simulink model "zynqRadioWLAN80211BeaconRxFPGAAD9361AD9364SL"  (R2016a)
settings: Solver=FixedStepDiscrete  SolverMode=SingleTasking  StartTime=0.0  StopTime=inf  RelTol=1e-3
PreLoadFcn:
  | load('commwlan80211BusTypes')
  | openMPDUGUI = true;
PostLoadFcn:
  | zynqRadioWLAN80211BeaconRxFPGAAD9361AD9364SL_params('init')
  | zynqRadioWLAN80211BeaconRxFPGAAD9361AD9364SL_params('scope')
InitFcn:
  | load('commwlan80211BusTypes')
  | openMPDUGUI = true;
  | mpduFigPos= [ 100 100 400 500];
model workspace: external: MAT-File (data not in the file)
undefined symbols (not defined in the file or in its folder): F, p80211, p80211hdl
libraries: simulink x11, hdlsllib x4, commutil2 x3, commwlan80211BeaconLib x2, commdigbbndpm3 x1, commsequence2 x1, commcrc2 x1, dspstat3 x1, dspmlti4 x1, dspsigops x1, dspmathops x1, sdrzblksprivate x1
(part 1 of 2)
CloseFcn:
  | clear BeaconFrameBodyType BeaconMPDUType CapabilityType FrameCtrlType InfoElementType MPDUHeaderType p80211 commwlan80211TxFilt rcvd openMPDUGUI mpduFigPos p80211hdl Hd
  | hFig = findall(0, 'Type', 'figure', 'Name', '802.11 Beacon Frame');
  | if ishghandle(hFig)
  | close(hFig);
  | end
  | clear hFig
  | if (exist('ans')==1) && (iscell(ans) && (numel(ans) == 0))
  | clear ans
  | end
Description:
  | IEEE 802.11 WLAN Beacon Frame Receiver for Captured Data
  | 
  | This example shows how to process a captured beacon frame and display the
  | frame information.
settings Model: ModifiedByFormat=The MathWorks Inc.  SimulationMode=accelerator  ExtModeTrigDuration=100  Creator=The MathWorks, Inc.  LastModifiedBy=The MathWorks Inc.
settings DataIOCC: LimitDataPoints=on  SaveFormat=Array  SaveOutput=off  SignalLogging=off  DSMLogging=off  StateSaveName=tmp_raccel_xout
settings OptimizationCC: BlockReduction=off  ConditionallyExecuteInputs=off  DefaultParameterBehavior=Inlined  InlineInvariantSignals=on  ExpressionDepthLimit=2147483647  EfficientMapNaN2IntZero=off
settings DebuggingCC: ReadBeforeWriteMsg=DisableAll  WriteAfterWriteMsg=DisableAll  WriteAfterReadMsg=DisableAll  AlgebraicLoopMsg=error  UnderspecifiedInitializationDetection=Classic  MergeDetectMultiDrivingBlocksExec=none  SolverPrmCheckMsg=warning  InheritedTsInSrcMsg=none  SingleTaskRateTransMsg=error  IntegerOverflowMsg=none  ParameterDowncastMsg=none  ParameterOverflowMsg=none  ParameterPrecisionLossMsg=none  ParameterTunabilityLossMsg=none  UniqueDataStoreMsg=error  AllowSymbolicDim=off  ModelReferenceDataLoggingMessage=none  StateNameClashWarn=warning  IntegerSaturationMsg=none
settings HardwareCC: ProdBitPerPointer=32  ProdLargestAtomicFloat=None  ProdIntDivRoundTo=Undefined  ProdEndianess=Unspecified  ProdWordSize=32  ProdHWDeviceType=ASIC/FPGA->ASIC/FPGA  TargetBitPerPointer=64  TargetLongLongMode=on  TargetIntDivRoundTo=Zero  TargetEndianess=LittleEndian  TargetWordSize=64  TargetHWDeviceType=MATLAB Host  ProdEqTarget=off
settings ModelReferenceCC: PropagateSignalLabelsOutOfModel=off
settings RTWCC: SystemTargetFile=raccel.tlc  TemplateMakefile=raccel_default_tmf  RTWVerbose=off  RTWUseSimCustomCode=on
settings CodeAppCC: GenerateComments=off  MaxIdLength=128  MangleLength=10  SimulinkBlockComments=off
settings RaccelTargetCC: ERTMultiwordTypeDef=System defined  ERTMultiwordLength=256  ParMdlRefBuildCompliant=off  GeneratePreprocessorConditionals=Disable all  ERTFirstTimeCompliant=off  MultiInstanceERTCode=off  ENABLE_SLEXEC_SSBRIDGE=0  RTWCAPISignals=off  RTWCAPIParams=off
settings ConfigComp: CovModelRefEnable=Off  CovSFcnEnable=off

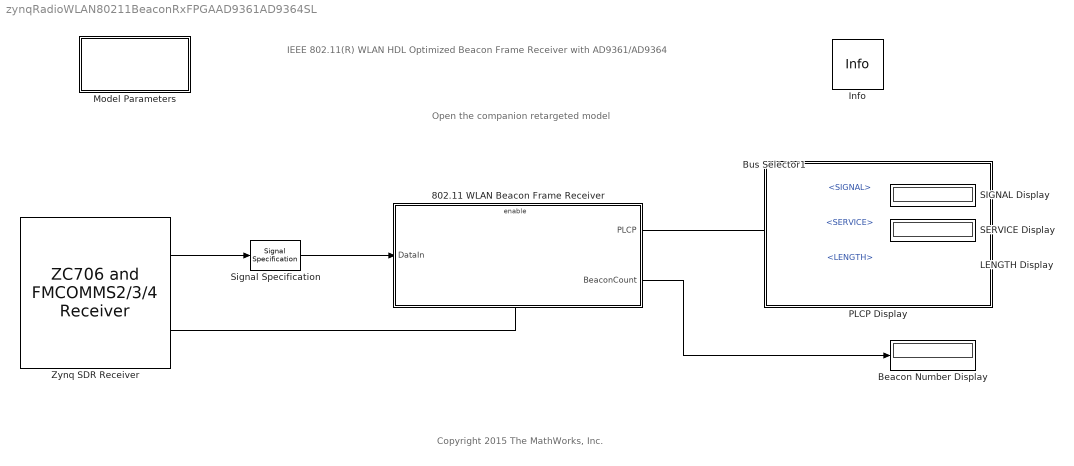
== system zynqRadioWLAN80211BeaconRxFPGAAD9361AD9364SL ==
  note: IEEE 802.11(R) WLAN
      | HDL Optimized Beacon Frame Receiver with AD9361/AD9364
  note: Copyright 2015 The MathWorks, Inc.
  note: Open the companion retargeted model
  802.11 WLAN Beacon Frame Receiver : Subsystem
  Beacon Number Display : Display
  Bus Selector1 : BusSelector  OutputSignals=SIGNAL,SERVICE,LENGTH
  Info : sdrzblksprivate/Info  SystemSampleTime=-1
  LENGTH Display : Display
  Model Parameters : Subsystem  mask(Model Parameters){chanNum=1, rfGain=30, rfFreqOffset=0, agcLoopGain=0.05, agcMaxGain=400, corrThreshold=1400}
      mask prompts: chanNum "Channel number"; rfGain "RF board gain:"; rfFreqOffset "RF center frequency offset:"; agcLoopGain "AGC loop gain:"; agcMaxGain "Maximum AGC gain:"; corrThreshold "Synchronization threshold:"
      mask help:
      | Choose 802.11 receiver parameters.
      |
      | You can select channel number for the 802.11 signals. You can set the AGC parameters and samples per chip used in the receiver. You can also set the synchronization threshold value to determine the correlation threshold used to declare the presence of an 802.11 packet.
      mask init:
      | zynqRadioWLAN80211BeaconRxFPGAAD9361AD9364SL_params('init', ...
      |     'ChannelNumber',   chanNum, ...
      |     'AGCLoopGain',     agcLoopGain, ...
      |     'AGCMaxGain',      agcMaxGain, ...
      |     'CorrThreshold',   corrThreshold, ...
      |     'RadioGain',       rfGain, ...
      |     'RadioFreqOffset', rfFreqOffset ...
      |     );
      mask TypeOptions chanNum: 1 | 2 | 3 | 4 | 5 | 6 | 7 | 8 | 9 | 10 | 11
      mask Display: disp('Model\nParameters')
  PLCP Display : Subsystem
      mask Display: disp('')
  SERVICE Display : Display
      settings: Format=hex (Stored Integer)
  SIGNAL Display : Display
      settings: Format=hex (Stored Integer)
  Signal Specification : SignalSpecification  SampleTime=p80211.RadioFrameLength/p80211.RadioBasebandRate
  Zynq SDR Receiver : zc706fmc234_lib/ZC706 and  FMCOMMS2//3//4  Receiver  IPAddress=192.168.3.2  CenterFrequencySource=Dialog  CenterFrequency=2.412e9+(p80211.ChannelNumber-1)*5e6+p80211.RadioFreqOffset  GainSource=Dialog  Gain=p80211.RadioGain  ChannelMapping=1  BasebandSampleRate=p80211.RadioBasebandRate  EnableBurstMode=on  NumFramesInBurst=p80211.RadioNumFramesInBurst  OutputDataType=int16  SamplesPerFrame=p80211.RadioFrameLength  LostSamplesOutputPort=off  RSSIOutputPort=off  DMATimeoutValue=1  blockMode=Normal  EnableQuadratureTracking=on  EnableRFDCTracking=on  EnableBasebandDCTracking=on  BypassUserLogic=on  ShowAdvancedProperties=on  ShowInternalProperties=off  subDeviceList=zynqReceiver  sdrExecutionMode=HW  dataUDPPort=-1  ctrlUDPPort=-1  SourceSelect=RF data  SourceConfiguration1=1023  FIRCoefficientSize=[ 128; 128 ]  FIRCoefficients=[ 111, -87, 147, -127, -18, -286, -312, -555, -601, -722, -642, -555, -303, -66, 221, 393, 488, 403, 219, -74, -343, -550, -582, -450, -146, 221, 569, 759, 735, 463, 20, -487, -885, -1048, -883, -418, 243, 897, 1340, 1394, 1002, 228, -715, -1549, -1980, -1819, -1028, 217, 1583, 2635, 2980, 2377, 853, -1275, -3435, -4926, -5080, -3454, 40, 5065, 10903, 16581, 21085, 23573, 23573, 21085, 16581, 10903, 5065, 40, -3454, -5080, -4926, -3435, -1275, 853, 2377, 2980, 2635, 1583, 217, -1028, -1819, -1980, -1549, -715, 228, 1002, 1394, 1340, 897, 243, -418, -883, -1048, -885, -487, 20, 463, 735, 759, 569, 221, -146, -450, -582, -550, -343, -74, 219, 403, 488, 393, 221, -66, -303, -555, -642, -722, -601, -555, -312, -286, -18, -127, 147, -87, 111; 382, -200, 711, -41, 645, 36, 346, -194, -119, -543, -472, -646, -404, -312, 45, 197, 413, 346, 241, -93, -373, -680, -755, -689, -356, 51, 515, 795, 870, 609, 136, -488, -1009, -1303, -1191, -712, 69, 885, 1516, 1692, 1336, 468, -662, -1740, -2378, -2329, -1494, -55, 1620, 2995, 3584, 3045, 1368, -1121, -3755, -5708, -6156, -4542, -710, 4969, 11669, 18243, 23486, 26391, 26391, 23486, 18243, 11669, 4969, -710, -4542, -6156, -5708, -3755, -1121, 1368, 3045, 3584, 2995, 1620, -55, -1494, -2329, -2378, -1740, -662, 468, 1336, 1692, 1516, 885, 69, -712, -1191, -1303, -1009, -488, 136, 609, 870, 795, 515, 51, -356, -689, -755, -680, -373, -93, 241, 346, 413, 197, 45, -312, -404, -646, -472, -543, -119, -194, 346, 36, 645, -41, 711, -200, 382 ]  FIRGain=[ 0; -12 ]  FIRDecimInterpFactor=[ 4; 4 ]  AnalogFilterCutoff=[ 2560000; 2560000 ]  FilterPathRates=[ 737280000, 184320000, 61440000, 30720000, 15360000, 3840000; 737280000, 184320000, 61440000, 30720000, 15360000, 3840000 ]  FilterDesignTypeForTx=DefaultFilterFromOther  FilterDesignTypeForRx=DefaultFilter  BISTLoopbackConfig=No Loopback  BISTPRBSMode=PRBS Disable  BISTToneMode=Tone Disable  BISTToneFrequency=F/32  BISTToneLevel=-6  BISTChannelMask=0  DataIsComplex=on  SimulateUsing=Code generation
  wires:
  802.11 WLAN Beacon Frame Receiver/1(PLCP) -> Bus Selector1/1
  Bus Selector1/3 -> LENGTH Display/1  "<LENGTH>"
  Bus Selector1/1 -> SIGNAL Display/1  "<SIGNAL>"
  Bus Selector1/2 -> SERVICE Display/1  "<SERVICE>"
  Zynq SDR Receiver/1 -> Signal Specification/1
  Zynq SDR Receiver/2 -> 802.11 WLAN Beacon Frame Receiver/Enable
  Signal Specification/1 -> 802.11 WLAN Beacon Frame Receiver/1(DataIn)
  802.11 WLAN Beacon Frame Receiver/2(BeaconCount) -> Beacon Number Display/1

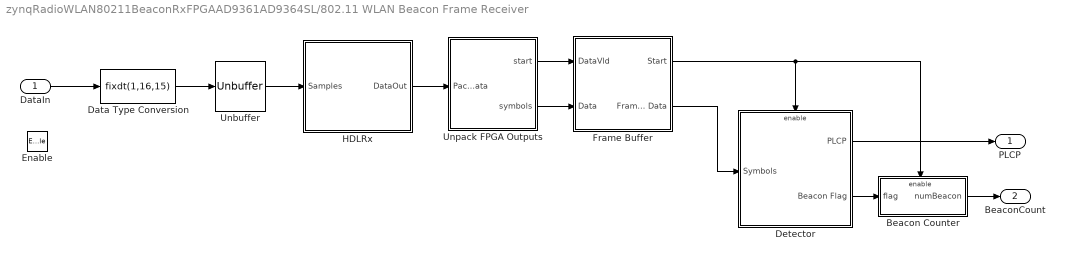
== system zynqRadioWLAN80211BeaconRxFPGAAD9361AD9364SL/802.11 WLAN Beacon Frame Receiver ==
  DataIn : Inport
  Enable : EnablePort
  Beacon Counter : Subsystem
  Data Type Conversion : DataTypeConversion  OutDataTypeStr=fixdt(1,16,15)  ConvertRealWorld=Stored Integer (SI)
  Detector : Subsystem
      settings: CloseFcn=clear BeaconFrameBodyType rcvd
  Frame Buffer : Subsystem
  HDLRx : Subsystem
  Unbuffer : Unbuffer  SampleBasedProcessing=Same as frame based
  Unpack FPGA Outputs : Subsystem
  PLCP : Outport
  BeaconCount : Outport  Port=2
  wires:
  Frame Buffer/1(Start) -> Detector/Enable, Beacon Counter/Enable
  Unbuffer/1 -> HDLRx/1(Samples)
  Frame Buffer/2(Framed Data) -> Detector/1(Symbols)
  Beacon Counter/1(numBeacon) -> BeaconCount/1
  Data Type Conversion/1 -> Unbuffer/1
  Detector/1(PLCP) -> PLCP/1
  DataIn/1 -> Data Type Conversion/1
  Detector/2(Beacon Flag) -> Beacon Counter/1(flag)
  HDLRx/1(DataOut) -> Unpack FPGA Outputs/1(PackedData)
  Unpack FPGA Outputs/1(start) -> Frame Buffer/1(DataVld)
  Unpack FPGA Outputs/2(symbols) -> Frame Buffer/2(Data)

== system zynqRadioWLAN80211BeaconRxFPGAAD9361AD9364SL/Model Parameters ==

== system zynqRadioWLAN80211BeaconRxFPGAAD9361AD9364SL/PLCP Display ==

== system zynqRadioWLAN80211BeaconRxFPGAAD9361AD9364SL/802.11 WLAN Beacon Frame Receiver/Beacon Counter ==
  flag : Inport
  Enable : EnablePort
  MATLAB Function : MATLAB Function  TreatAsAtomicUnit=on
  numBeacon : Outport
  wires:
  MATLAB Function/1(numBeacon) -> numBeacon/1
  flag/1 -> MATLAB Function/1(beaconflag)

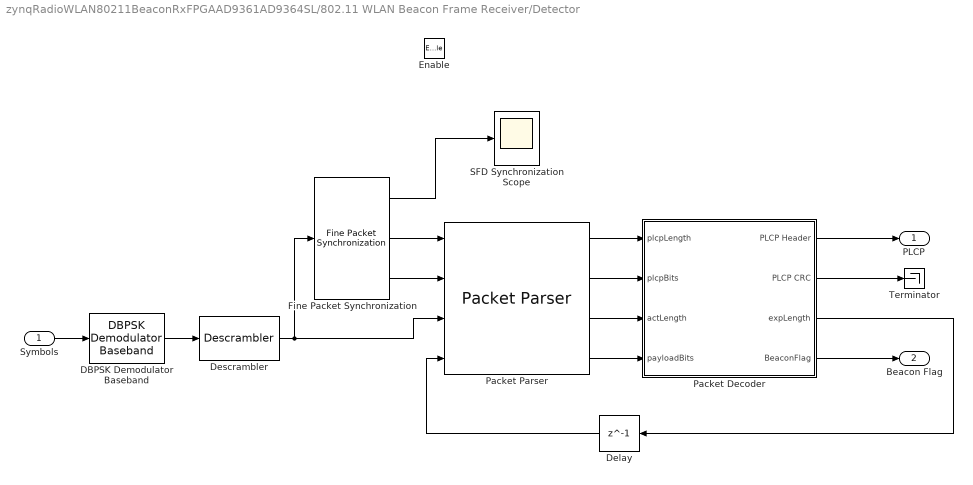
== system zynqRadioWLAN80211BeaconRxFPGAAD9361AD9364SL/802.11 WLAN Beacon Frame Receiver/Detector ==
  Symbols : Inport
  Enable : EnablePort  StatesWhenEnabling=reset  PropagateVarSize=During execution
  DBPSK Demodulator Baseband : commdigbbndpm3/DBPSK Demodulator Baseband  Ph=0  outDtype=uint32
  Delay : Delay  DelayLength=1  InitialCondition=0  InputProcessing=Columns as channels (frame based)
  Descrambler : commsequence2/Descrambler  M=2  poly=p80211.ScramblerPolynomial  iniStaSource=Dialog Parameter  ini_sta=[0 0 0 0 0 0 0]  resetViaPort=off
  Fine Packet Synchronization : commwlan80211BeaconLib/Fine Packet Synchronization
  Packet Decoder : Subsystem
  Packet Parser : commwlan80211BeaconLib/Packet Parser
  SFD Synchronization Scope : Scope
      settings: Priority=10
  Terminator : Terminator
  PLCP : Outport
  Beacon Flag : Outport  Port=2  InitialOutput=1
  wires:
  Fine Packet Synchronization/1 -> SFD Synchronization Scope/1
  DBPSK Demodulator Baseband/1 -> Descrambler/1
  Symbols/1 -> DBPSK Demodulator Baseband/1
  Descrambler/1 -> Fine Packet Synchronization/1, Packet Parser/3
  Fine Packet Synchronization/2 -> Packet Parser/1
  Fine Packet Synchronization/3 -> Packet Parser/2
  Delay/1 -> Packet Parser/4
  Packet Parser/2 -> Packet Decoder/2(plcpBits)
  Packet Parser/3 -> Packet Decoder/3(actLength)
  Packet Parser/4 -> Packet Decoder/4(payloadBits)
  Packet Decoder/1(PLCP Header) -> PLCP/1
  Packet Parser/1 -> Packet Decoder/1(plcpLength)
  Packet Decoder/2(PLCP CRC) -> Terminator/1
  Packet Decoder/3(expLength) -> Delay/1
  Packet Decoder/4(BeaconFlag) -> Beacon Flag/1

== system zynqRadioWLAN80211BeaconRxFPGAAD9361AD9364SL/802.11 WLAN Beacon Frame Receiver/Frame Buffer ==
  DataVld : Inport
  Data : Inport  Port=2
  Buffer1 : Buffer  N=128  TreatMby1Signals=One channel  OutputFrames=off
  Buffer2 : Buffer  N=128  TreatMby1Signals=One channel  OutputFrames=off
  Data Type Conversion : DataTypeConversion
  Received Symbols : ConstellationDiagram  Tag=ScatterPlot  Priority=2
  data_framer : MATLAB Function  TreatAsAtomicUnit=on
  Start : Outport
  Framed Data : Outport  Port=2
  wires:
  Data Type Conversion/1 -> Framed Data/1
  data_framer/2(framed_data) -> Data Type Conversion/1
  data_framer/1(RxGo) -> Start/1
  Buffer1/1 -> data_framer/2(data), Received Symbols/1
  DataVld/1 -> Buffer2/1
  Data/1 -> Buffer1/1
  Buffer2/1 -> data_framer/1(datavld)

== system zynqRadioWLAN80211BeaconRxFPGAAD9361AD9364SL/802.11 WLAN Beacon Frame Receiver/HDLRx ==
  Samples : Inport
  FPGA to Host : Subsystem
  HDLRx Controller : Subsystem
  HDLRx Front End : Subsystem
  DataOut : Outport
  wires:
  Samples/1 -> HDLRx Front End/1(Samples)
  HDLRx Controller/1(Start) -> FPGA to Host/1(start)
  HDLRx Front End/1(rcvd) -> HDLRx Controller/1(Rx Signal)
  HDLRx Controller/2(Symbols) -> FPGA to Host/2(symbol)
  FPGA to Host/1(Out) -> DataOut/1

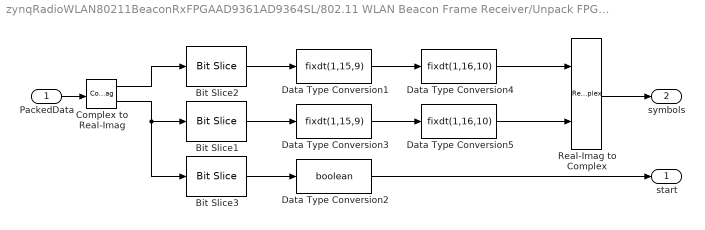
== system zynqRadioWLAN80211BeaconRxFPGAAD9361AD9364SL/802.11 WLAN Beacon Frame Receiver/Unpack FPGA Outputs ==
  PackedData : Inport
  Bit Slice1 : hdlsllib/HDL Operations/Bit Slice  lidx=15  ridx=1
  Bit Slice2 : hdlsllib/HDL Operations/Bit Slice  lidx=15  ridx=1
  Bit Slice3 : hdlsllib/HDL Operations/Bit Slice  lidx=0  ridx=0
  Complex to Real-Imag : ComplexToRealImag
  Data Type Conversion1 : DataTypeConversion  OutDataTypeStr=fixdt(1,15,9)  ConvertRealWorld=Stored Integer (SI)
  Data Type Conversion2 : DataTypeConversion  OutDataTypeStr=boolean
  Data Type Conversion3 : DataTypeConversion  OutDataTypeStr=fixdt(1,15,9)  ConvertRealWorld=Stored Integer (SI)
  Data Type Conversion4 : DataTypeConversion  OutDataTypeStr=fixdt(1,16,10)
  Data Type Conversion5 : DataTypeConversion  OutDataTypeStr=fixdt(1,16,10)
  Real-Imag to Complex : RealImagToComplex
  start : Outport
  symbols : Outport  Port=2
  wires:
  PackedData/1 -> Complex to Real-Imag/1
  Real-Imag to Complex/1 -> symbols/1
  Complex to Real-Imag/1 -> Bit Slice2/1
  Complex to Real-Imag/2 -> Bit Slice3/1, Bit Slice1/1
  Bit Slice3/1 -> Data Type Conversion2/1
  Data Type Conversion2/1 -> start/1
  Bit Slice2/1 -> Data Type Conversion1/1
  Bit Slice1/1 -> Data Type Conversion3/1
  Data Type Conversion1/1 -> Data Type Conversion4/1
  Data Type Conversion4/1 -> Real-Imag to Complex/1
  Data Type Conversion3/1 -> Data Type Conversion5/1
  Data Type Conversion5/1 -> Real-Imag to Complex/2

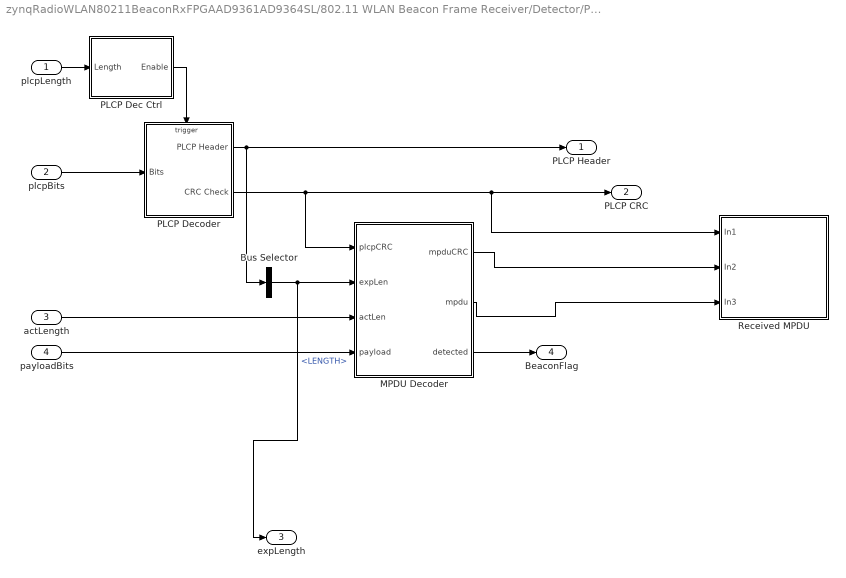
== system zynqRadioWLAN80211BeaconRxFPGAAD9361AD9364SL/802.11 WLAN Beacon Frame Receiver/Detector/Packet Decoder ==
  plcpLength : Inport
  plcpBits : Inport  Port=2
  actLength : Inport  Port=3
  payloadBits : Inport  Port=4
  Bus Selector : BusSelector  OutputSignals=LENGTH
  MPDU Decoder : MATLAB Function  TreatAsAtomicUnit=on
  PLCP Dec Ctrl : Subsystem
  PLCP Decoder : Subsystem
  Received MPDU : Subsystem  mask(MPDU GUI){OpenScopeAtSimStart=openMPDUGUI, figPosition=mpduFigPos}
      mask prompts: OpenScopeAtSimStart "Open GUI at start of simulation"; figPosition "Position"
      mask help: Display contents of the MPDU.
      mask Display: disp('MPDU GUI')
  PLCP Header : Outport
  PLCP CRC : Outport  Port=2
  expLength : Outport  Port=3
  BeaconFlag : Outport  Port=4
  wires:
  PLCP Dec Ctrl/1(Enable) -> PLCP Decoder/Trigger
  Bus Selector/1 -> MPDU Decoder/2(expLen), expLength/1  "<LENGTH>"
  PLCP Decoder/1(PLCP Header) -> Bus Selector/1, PLCP Header/1
  plcpLength/1 -> PLCP Dec Ctrl/1(Length)
  plcpBits/1 -> PLCP Decoder/1(Bits)
  actLength/1 -> MPDU Decoder/3(actLen)
  payloadBits/1 -> MPDU Decoder/4(payload)
  MPDU Decoder/1(mpduCRC) -> Received MPDU/2(In2)
  MPDU Decoder/2(mpdu) -> Received MPDU/3(In3)
  PLCP Decoder/2(CRC Check) -> MPDU Decoder/1(plcpCRC), Received MPDU/1(In1), PLCP CRC/1
  MPDU Decoder/3(detected) -> BeaconFlag/1

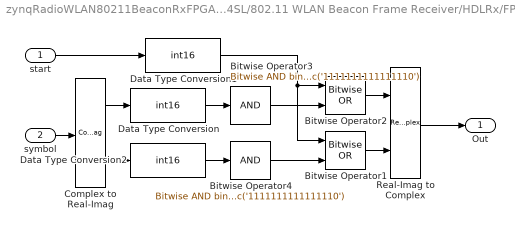
== system zynqRadioWLAN80211BeaconRxFPGAAD9361AD9364SL/802.11 WLAN Beacon Frame Receiver/HDLRx/FPGA to Host ==
  start : Inport
  symbol : Inport  Port=2
  Bitwise Operator1 : simulink/Logic and Bit Operations/Bitwise Operator  logicop=OR  UseBitMask=off  NumInputPorts=2  BitMask=bin2dec('11011001')  BitMaskRealWorld=Stored Integer
  Bitwise Operator2 : simulink/Logic and Bit Operations/Bitwise Operator  logicop=OR  UseBitMask=off  NumInputPorts=2  BitMask=bin2dec('11011001')  BitMaskRealWorld=Stored Integer
  Bitwise Operator3 : simulink/Logic and Bit Operations/Bitwise Operator  logicop=AND  UseBitMask=on  BitMask=bin2dec('1111111111111110')  BitMaskRealWorld=Stored Integer
  Bitwise Operator4 : simulink/Logic and Bit Operations/Bitwise Operator  logicop=AND  UseBitMask=on  BitMask=bin2dec('1111111111111110')  BitMaskRealWorld=Stored Integer
  Complex to Real-Imag : ComplexToRealImag
  Data Type Conversion : DataTypeConversion  OutDataTypeStr=int16  ConvertRealWorld=Stored Integer (SI)
  Data Type Conversion1 : DataTypeConversion  OutDataTypeStr=int16
  Data Type Conversion2 : DataTypeConversion  OutDataTypeStr=int16  ConvertRealWorld=Stored Integer (SI)
  Real-Imag to Complex : RealImagToComplex
  Out : Outport
  wires:
  symbol/1 -> Complex to Real-Imag/1
  start/1 -> Data Type Conversion1/1
  Bitwise Operator2/1 -> Real-Imag to Complex/1
  Bitwise Operator1/1 -> Real-Imag to Complex/2
  Real-Imag to Complex/1 -> Out/1
  Complex to Real-Imag/1 -> Data Type Conversion/1
  Complex to Real-Imag/2 -> Data Type Conversion2/1
  Data Type Conversion/1 -> Bitwise Operator3/1
  Data Type Conversion2/1 -> Bitwise Operator4/1
  Bitwise Operator4/1 -> Bitwise Operator1/2
  Bitwise Operator3/1 -> Bitwise Operator2/2
  Data Type Conversion1/1 -> Bitwise Operator1/1, Bitwise Operator2/1

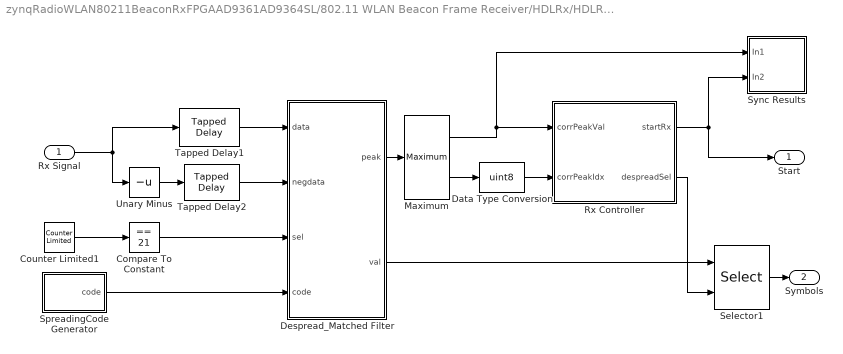
== system zynqRadioWLAN80211BeaconRxFPGAAD9361AD9364SL/802.11 WLAN Beacon Frame Receiver/HDLRx/HDLRx Controller ==
  Rx Signal : Inport
  Compare To Constant : simulink/Logic and Bit Operations/Compare To Constant  relop===  const=21  OutDataTypeStr=boolean
  Counter Limited1 : simulink/Sources/Counter Limited  uplimit=21  tsamp=-1
  Data Type Conversion : DataTypeConversion  OutDataTypeStr=uint8
  Despread_Matched Filter : Subsystem
  Maximum : dspstat3/Maximum  fcn=Value and Index  reset=None  InputProcessing=Columns as channels (frame based)  indexBase=One  operateOver=Each column  Dimension=1  operation=maximum  roiEnable=off  roiType=Rectangles  roiPortion=Entire ROI  roiOutput=Individual statistics for each ROI  roiFlag=off  accumDataTypeStr=Inherit: Same as product output  accumLastDataTypeStr=Inherit: Same as product output  roundingMode=Floor  overflowMode=off
  Rx Controller : MATLAB Function  TreatAsAtomicUnit=on
  Selector1 : Selector  InputPortWidth=22  IndexOptions=Index vector (port)  Indices=[1 3]  OutputSizes=1
  "SpreadingCode Generator " : Subsystem
  Sync Results : Subsystem
  Tapped Delay1 : simulink/Discrete/Tapped Delay  vinit=0  samptime=-1  NumDelays=21  DelayOrder=Newest  includeCurrent=on
  Tapped Delay2 : simulink/Discrete/Tapped Delay  vinit=0  samptime=-1  NumDelays=21  DelayOrder=Newest  includeCurrent=on
  Unary Minus : UnaryMinus
  Start : Outport
  Symbols : Outport  Port=2
  wires:
  Compare To Constant/1 -> Despread_Matched Filter/3(sel)
  Despread_Matched Filter/2(val) -> Selector1/1
  Despread_Matched Filter/1(peak) -> Maximum/1
  Rx Signal/1 -> Tapped Delay1/1, Unary Minus/1
  Tapped Delay1/1 -> Despread_Matched Filter/1(data)
  Selector1/1 -> Symbols/1
  Rx Controller/2(despreadSel) -> Selector1/2
  Maximum/1 -> Sync Results/1(In1), Rx Controller/1(corrPeakVal)
  Counter Limited1/1 -> Compare To Constant/1
  Unary Minus/1 -> Tapped Delay2/1
  Tapped Delay2/1 -> Despread_Matched Filter/2(negdata)
  Maximum/2 -> Data Type Conversion/1
  Data Type Conversion/1 -> Rx Controller/2(corrPeakIdx)
  Rx Controller/1(startRx) -> Start/1, Sync Results/2(In2)
  "SpreadingCode Generator "/1(code) -> Despread_Matched Filter/4(code)

== system zynqRadioWLAN80211BeaconRxFPGAAD9361AD9364SL/802.11 WLAN Beacon Frame Receiver/HDLRx/HDLRx Front End ==
  note: AGC implements the square law method:
      | e(n) = R - abs(x(n))^2;  % R = 1;
      | g(n) = g(n-1) + K*e(n);
  note: |U|^2 = re(u)^2+im(u)^2
  Samples : Inport
  AGC : Subsystem
  AGC Results : Subsystem
  Coarse Frequency Compensation : Subsystem
  Delay3 : Delay  DelayLength=1  InitialCondition=0
  Frequency Offset : Scope
  Inputreg : Delay  DelayLength=1  InitialCondition=0
  RCFilter : Subsystem
  rcvd : Outport
  wires:
  AGC/2(gain) -> AGC Results/2(In2)
  RCFilter/1(Out1) -> Delay3/1
  Samples/1 -> Inputreg/1
  Inputreg/1 -> RCFilter/1(In1)
  Delay3/1 -> AGC/1(x), AGC Results/3(In3)
  AGC/1(y) -> Coarse Frequency Compensation/1(x), AGC Results/1(In1)
  Coarse Frequency Compensation/1(y) -> rcvd/1
  Coarse Frequency Compensation/2(offset) -> Frequency Offset/1

== system zynqRadioWLAN80211BeaconRxFPGAAD9361AD9364SL/802.11 WLAN Beacon Frame Receiver/Detector/Packet Decoder/PLCP Dec Ctrl ==
  Length : Inport
  Compare To Constant : simulink/Logic and Bit Operations/Compare To Constant  relop=>=  const=p80211.PLCPHeaderLength  OutDataTypeStr=uint8
  Enable : Outport
  wires:
  Length/1 -> Compare To Constant/1
  Compare To Constant/1 -> Enable/1

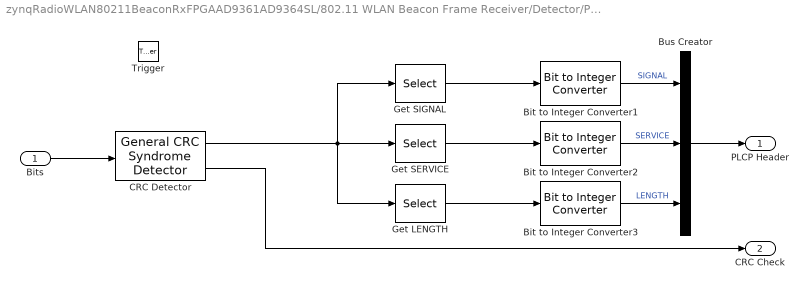
== system zynqRadioWLAN80211BeaconRxFPGAAD9361AD9364SL/802.11 WLAN Beacon Frame Receiver/Detector/Packet Decoder/PLCP Decoder ==
  Bits : Inport
  Trigger : TriggerPort  VariantControl=Variant  PortDimensions=1
  Bit to Integer Converter1 : commutil2/Bit to Integer Converter  nbits=8  bitOrder=LSB first  signedOutputValues=Unsigned  outDtype=Inherit via internal rule  outDtypeSigned=Inherit via internal rule
  Bit to Integer Converter2 : commutil2/Bit to Integer Converter  nbits=8  bitOrder=LSB first  signedOutputValues=Unsigned  outDtype=Inherit via internal rule  outDtypeSigned=Inherit via internal rule
  Bit to Integer Converter3 : commutil2/Bit to Integer Converter  nbits=16  bitOrder=LSB first  signedOutputValues=Unsigned  outDtype=uint16  outDtypeSigned=Inherit via internal rule
  Bus Creator : BusCreator  Inputs=3
  CRC Detector : commcrc2/General CRC Syndrome Detector  genPoly=[1 0 0 0 1 0 0 0 0 0 0 1 0 0 0 0 1]  iniStates=1  directMethod=on  reflectInputBytes=off  reflectChecksums=off  finalXOR=1  numChecksums=1
  Get LENGTH : Selector  InputPortWidth=32  IndexOptions=Index vector (dialog)  Indices=17:32  OutputSizes=1
  Get SERVICE : Selector  InputPortWidth=32  IndexOptions=Index vector (dialog)  Indices=9:16  OutputSizes=1
  Get SIGNAL : Selector  InputPortWidth=32  IndexOptions=Index vector (dialog)  Indices=1:8  OutputSizes=1
  PLCP Header : Outport
  CRC Check : Outport  Port=2
  wires:
  Bus Creator/1 -> PLCP Header/1
  Bit to Integer Converter3/1 -> Bus Creator/3  "LENGTH"
  Bits/1 -> CRC Detector/1
  Bit to Integer Converter2/1 -> Bus Creator/2  "SERVICE"
  Bit to Integer Converter1/1 -> Bus Creator/1  "SIGNAL"
  Get LENGTH/1 -> Bit to Integer Converter3/1
  Get SERVICE/1 -> Bit to Integer Converter2/1
  Get SIGNAL/1 -> Bit to Integer Converter1/1
  CRC Detector/1 -> Get SIGNAL/1, Get SERVICE/1, Get LENGTH/1
  CRC Detector/2 -> CRC Check/1

== system zynqRadioWLAN80211BeaconRxFPGAAD9361AD9364SL/802.11 WLAN Beacon Frame Receiver/Detector/Packet Decoder/Received MPDU ==
  In1 : Inport
  In2 : Inport  Port=2
  In3 : Inport  Port=3
  Received MPDU GUI : MATLAB Function  TreatAsAtomicUnit=on
  wires:
  In3/1 -> Received MPDU GUI/3(mpdu)
  In2/1 -> Received MPDU GUI/2(mpduCRC)
  In1/1 -> Received MPDU GUI/1(plcpCRC)

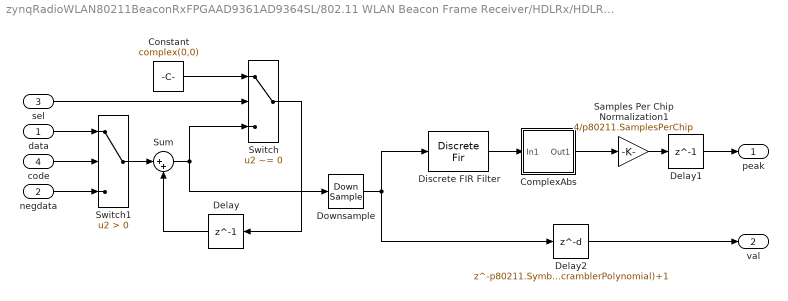
== system zynqRadioWLAN80211BeaconRxFPGAAD9361AD9364SL/802.11 WLAN Beacon Frame Receiver/HDLRx/HDLRx Controller/Despread_Matched Filter ==
  data : Inport
  negdata : Inport  Port=2
  sel : Inport  Port=3
  code : Inport  Port=4
  ComplexAbs : Subsystem
  Constant : Constant  Value=complex(0,0)  OutDataTypeStr=fixdt(1,16,7)  SampleTime=-1
  Delay : Delay  DelayLength=1  InitialCondition=0
  Delay1 : Delay  DelayLength=1  InitialCondition=0
  Delay2 : Delay  DelayLength=p80211.SymbolsPerChannelFrame-2+length(p80211.ScramblerPolynomial)+1  InitialCondition=0
  Discrete FIR Filter : DiscreteFir  Coefficients=fliplr(reshape(p80211hdl.syncsig128,1,128))  CoefDataTypeStr=fixdt(1,4,0)  ProductDataTypeStr=fixdt(1,16,3)  AccumDataTypeStr=fixdt(1,16,2)
  Downsample : DownSample  N=22  phase=21  RateOptions=Allow multirate processing
  Samples Per Chip Normalization1 : Gain  Gain=4/p80211.SamplesPerChip  OutDataTypeStr=Inherit: Same as input
  Sum : Sum  Inputs=|++  OutDataTypeStr=fixdt(1,16,8)  RndMeth=Round  SaturateOnIntegerOverflow=on
  Switch : Switch  Criteria=u2 ~= 0
  Switch1 : Switch  Criteria=u2 > Threshold
  peak : Outport
  val : Outport  Port=2
  wires:
  sel/1 -> Switch/2
  Switch1/1 -> Sum/1
  Samples Per Chip Normalization1/1 -> Delay1/1
  Discrete FIR Filter/1 -> ComplexAbs/1(In1)
  ComplexAbs/1(Out1) -> Samples Per Chip Normalization1/1
  Downsample/1 -> Delay2/1, Discrete FIR Filter/1
  Delay2/1 -> val/1
  Switch/1 -> Delay/1
  Constant/1 -> Switch/1
  code/1 -> Switch1/2
  Delay/1 -> Sum/2
  data/1 -> Switch1/1
  Sum/1 -> Switch/3, Downsample/1
  negdata/1 -> Switch1/3
  Delay1/1 -> peak/1

== system zynqRadioWLAN80211BeaconRxFPGAAD9361AD9364SL/802.11 WLAN Beacon Frame Receiver/HDLRx/HDLRx Controller/SpreadingCode Generator  ==
  Selector : Selector  InputPortWidth=22  IndexOptions=Index vector (dialog)  Indices=1  OutputSizes=1
  Signal Specification1 : SignalSpecification  OutDataTypeStr=fixdt(1,2,0)
  Tapped Delay : simulink/Discrete/Tapped Delay  vinit=p80211hdl.spreadingcode  samptime=-1  NumDelays=22  DelayOrder=Oldest  includeCurrent=off
  code : Outport
  wires:
  Selector/1 -> code/1, Signal Specification1/1
  Signal Specification1/1 -> Tapped Delay/1
  Tapped Delay/1 -> Selector/1

== system zynqRadioWLAN80211BeaconRxFPGAAD9361AD9364SL/802.11 WLAN Beacon Frame Receiver/HDLRx/HDLRx Controller/Sync Results ==
  In1 : Inport
  In2 : Inport  Port=2
  Buffer : Buffer  N=p80211.SamplesPerChannelFrame  TreatMby1Signals=One channel  OutputFrames=off
  Buffer1 : Buffer  N=128  TreatMby1Signals=One channel  OutputFrames=off
  Synchronization Scope : Scope  NumInputPorts=2
      settings: Priority=1
  wires:
  In1/1 -> Buffer/1
  In2/1 -> Buffer1/1
  Buffer/1 -> Synchronization Scope/1
  Buffer1/1 -> Synchronization Scope/2

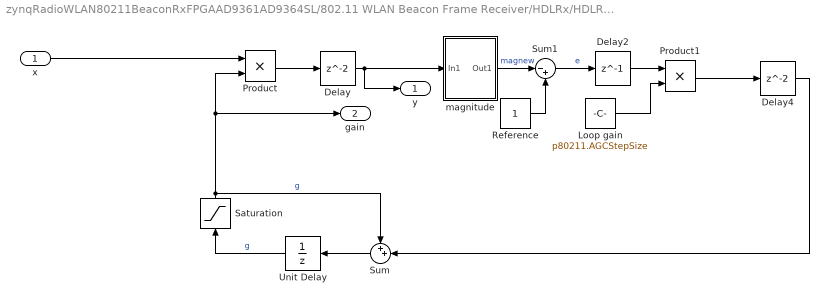
== system zynqRadioWLAN80211BeaconRxFPGAAD9361AD9364SL/802.11 WLAN Beacon Frame Receiver/HDLRx/HDLRx Front End/AGC ==
  x : Inport
  Delay : Delay  InitialCondition=0
  Delay2 : Delay  DelayLength=1  InitialCondition=0
  Delay4 : Delay  InitialCondition=0
  Loop gain : Constant  Value=p80211.AGCStepSize  OutDataTypeStr=fixdt(1,16,12)  SampleTime=-1
  Product : Product  OutDataTypeStr=fixdt(1,16,10)  SaturateOnIntegerOverflow=on
  Product1 : Product  OutDataTypeStr=fixdt(1,16,10)  SaturateOnIntegerOverflow=on
  Reference : Constant  OutDataTypeStr=fixdt(1,16,7)  SampleTime=-1
  Saturation : Saturate  UpperLimit=p80211.AGCUpperLimit  LowerLimit=1e-5  OutDataTypeStr=fixdt(1,16,6)
  Sum : Sum  Inputs=++|  OutDataTypeStr=fixdt(1,16,6)  SaturateOnIntegerOverflow=on
  Sum1 : Sum  Inputs=|-+  OutDataTypeStr=Inherit: Same as first input
  Unit Delay : UnitDelay  InitialCondition=1  SampleTime=-1
  magnitude : Subsystem
  y : Outport  PortDimensions=1
  gain : Outport  Port=2
  wires:
  x/1 -> Product/1
  Delay/1 -> y/1, magnitude/1(In1)
  Saturation/1 -> gain/1, Product/2, Sum/1  "g"
  Delay2/1 -> Product1/1
  Unit Delay/1 -> Saturation/1  "g"
  Loop gain/1 -> Product1/2
  Sum/1 -> Unit Delay/1
  Reference/1 -> Sum1/2
  Delay4/1 -> Sum/2
  magnitude/1(Out1) -> Sum1/1  "magnew"
  Product/1 -> Delay/1
  Product1/1 -> Delay4/1
  Sum1/1 -> Delay2/1  "e"

== system zynqRadioWLAN80211BeaconRxFPGAAD9361AD9364SL/802.11 WLAN Beacon Frame Receiver/HDLRx/HDLRx Front End/AGC Results ==
  In1 : Inport
  In2 : Inport  Port=2
  In3 : Inport  Port=3
  AGC Scope : Scope  NumInputPorts=3
  Buffer1 : Buffer  N=p80211.SamplesPerChannelFrame  TreatMby1Signals=One channel  OutputFrames=off
  Buffer2 : Buffer  N=p80211.SamplesPerChannelFrame  TreatMby1Signals=One channel  OutputFrames=off
  Buffer3 : Buffer  N=p80211.SamplesPerChannelFrame  TreatMby1Signals=One channel  OutputFrames=off
  ToFixPt1 : DataTypeConversion  OutDataTypeStr=double
  ToFixPt2 : DataTypeConversion  OutDataTypeStr=double
  wires:
  In3/1 -> Buffer1/1
  In2/1 -> Buffer2/1
  In1/1 -> Buffer3/1
  Buffer1/1 -> AGC Scope/1
  Buffer2/1 -> ToFixPt1/1
  Buffer3/1 -> ToFixPt2/1
  ToFixPt2/1 -> AGC Scope/3
  ToFixPt1/1 -> AGC Scope/2

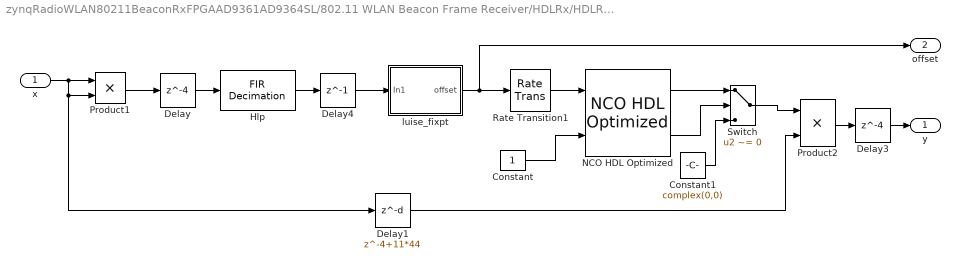
== system zynqRadioWLAN80211BeaconRxFPGAAD9361AD9364SL/802.11 WLAN Beacon Frame Receiver/HDLRx/HDLRx Front End/Coarse Frequency Compensation ==
  x : Inport  PortDimensions=1
  Constant : Constant  OutDataTypeStr=boolean  SampleTime=-1
  Constant1 : Constant  Value=complex(0,0)  OutDataTypeStr=fixdt(1,16,14)  SampleTime=-1
  Delay : Delay  DelayLength=4  InitialCondition=0
  Delay1 : Delay  DelayLength=4+11*44  InitialCondition=0
  Delay3 : Delay  DelayLength=4  InitialCondition=0
  Delay4 : Delay  DelayLength=1  InitialCondition=0
  Hlp : dspmlti4/FIR Decimation  Tag=BlockMethodSubSystem  FilterSource=Dialog parameters  h=Hd.Numerator  D=44  filtStruct=Direct form  FilterObject=Hd  framing=Allow multirate processing  inputOffset=0  outputBufInitCond=0  roundingMode=Floor  overflowMode=off  firstCoeffMode=Binary point scaling  firstCoeffWordLength=16  firstCoeffFracLength=15  firstCoeffDataTypeStr=fixdt(1,16,15)  firstCoeffMin=[]  firstCoeffMax=[]  firstCoeffLastDataTypeStr=fixdt(1,16,15)  prodOutputMode=Binary point scaling  prodOutputWordLength=32  prodOutputFracLength=20  prodOutputDataTypeStr=fixdt(1,32,20)  prodOutputLastDataTypeStr=fixdt(1,32,20)  accumDataTypeStr=Inherit: Same as product output  accumLastDataTypeStr=Inherit: Same as product output  outputMin=[]  outputMax=[]
  NCO HDL Optimized : dspsigops/NCO HDL Optimized  PhaseIncrementSource=Input port  PhaseIncrement=100  PhaseOffsetSource=Property  PhaseOffset=0  DitherSource=Property  NumDitherBits=4  PhaseQuantization=on  NumQuantizerAccumulatorBits=14  LUTCompress=on  ResetAction=off  ValidInputPort=on  Waveform=Complex exponential  PhasePort=off  AccumulatorWL=24  OutputDataType=Binary point scaling  OutputWL=16  OutputFL=14  SimulateUsing=Code generation
  Product1 : Product  OutDataTypeStr=fixdt(1,16,6)  RndMeth=Zero
  Product2 : Product  OutDataTypeStr=fixdt(1,16,10)  SaturateOnIntegerOverflow=on
  Rate Transition1 : RateTransition
  Switch : Switch  Criteria=u2 ~= 0
  luise_fixpt : Subsystem
  y : Outport
  offset : Outport  Port=2
  wires:
  Constant/1 -> NCO HDL Optimized/2
  NCO HDL Optimized/2 -> Switch/2
  x/1 -> Delay1/1, Product1/2, Product1/1
  Product1/1 -> Delay/1
  Product2/1 -> Delay3/1
  Delay/1 -> Hlp/1
  Delay3/1 -> y/1
  Hlp/1 -> Delay4/1
  Delay4/1 -> luise_fixpt/1(In1)
  Delay1/1 -> Product2/2
  Rate Transition1/1 -> NCO HDL Optimized/1
  luise_fixpt/1(offset) -> Rate Transition1/1, offset/1
  NCO HDL Optimized/1 -> Switch/1
  Constant1/1 -> Switch/3
  Switch/1 -> Product2/1

== system zynqRadioWLAN80211BeaconRxFPGAAD9361AD9364SL/802.11 WLAN Beacon Frame Receiver/HDLRx/HDLRx Front End/RCFilter ==
  In1 : Inport
  Discrete FIR Filter : DiscreteFir  FilterStructure=Direct form transposed  Coefficients=[0.0084136487845067817 -0.0012779096107435872 -0.023416382101133094 0.031830988618379061 0.040020036765270169 -0.10861435786336783 -0.053034100250923456 0.43511459293103077 0.76506964167771518 0.43511459293103077 -0.053034100250923456 -0.10861435786336783 0.040020036765270169 0.031830988618379061 -0.023416382101133094 -0.0012779096107435872 0.0084136487845067817]  CoefDataTypeStr=fixdt(1,16,15)  ProductDataTypeStr=fixdt(1,32,30)  AccumDataTypeStr=fixdt(1,32,29)  OutDataTypeStr=fixdt(1,16,15)
  Out1 : Outport
  wires:
  In1/1 -> Discrete FIR Filter/1
  Discrete FIR Filter/1 -> Out1/1

== system zynqRadioWLAN80211BeaconRxFPGAAD9361AD9364SL/802.11 WLAN Beacon Frame Receiver/HDLRx/HDLRx Controller/Despread_Matched Filter/ComplexAbs ==
  In1 : Inport
  Abs : Abs
  Abs1 : Abs
  Add7 : Sum  AccumDataTypeStr=fixdt(1,16,2)  OutDataTypeStr=Inherit: Same as first input
  Complex to Real-Imag : ComplexToRealImag
  Gain4 : Gain  Gain=0.4  OutDataTypeStr=fixdt(1,16,3)
  Relational Operator : RelationalOperator  OutDataTypeStr=boolean
  Switch : Switch  Criteria=u2 > Threshold
  Switch1 : Switch  Criteria=u2 > Threshold
  Out1 : Outport
  wires:
  In1/1 -> Complex to Real-Imag/1
  Abs/1 -> Switch/1, Switch1/3, Relational Operator/1
  Complex to Real-Imag/1 -> Abs/1
  Gain4/1 -> Add7/2
  Switch/1 -> Add7/1
  Switch1/1 -> Gain4/1
  Relational Operator/1 -> Switch/2, Switch1/2
  Abs1/1 -> Relational Operator/2, Switch/3, Switch1/1
  Add7/1 -> Out1/1
  Complex to Real-Imag/2 -> Abs1/1

== system zynqRadioWLAN80211BeaconRxFPGAAD9361AD9364SL/802.11 WLAN Beacon Frame Receiver/HDLRx/HDLRx Front End/AGC/magnitude ==
  note: http://www.dspguru.com/dsp/tricks/magnitude-estimator
  note: Frrekin book pp238
  In1 : Inport
  Complex to Real-Imag : ComplexToRealImag
  Delay : Delay  InitialCondition=0
  Delay1 : Delay  InitialCondition=0
  Product3 : Product  OutDataTypeStr=fixdt(1,16,7)  SaturateOnIntegerOverflow=on
  Product4 : Product  OutDataTypeStr=fixdt(1,16,7)  SaturateOnIntegerOverflow=on
  Sum1 : Sum  Inputs=|++  OutDataTypeStr=fixdt(1,16,7)  SaturateOnIntegerOverflow=on
  Out1 : Outport
  wires:
  Product3/1 -> Delay/1
  In1/1 -> Complex to Real-Imag/1
  Complex to Real-Imag/1 -> Product3/1, Product3/2
  Complex to Real-Imag/2 -> Product4/2, Product4/1
  Product4/1 -> Delay1/1
  Sum1/1 -> Out1/1
  Delay/1 -> Sum1/1
  Delay1/1 -> Sum1/2

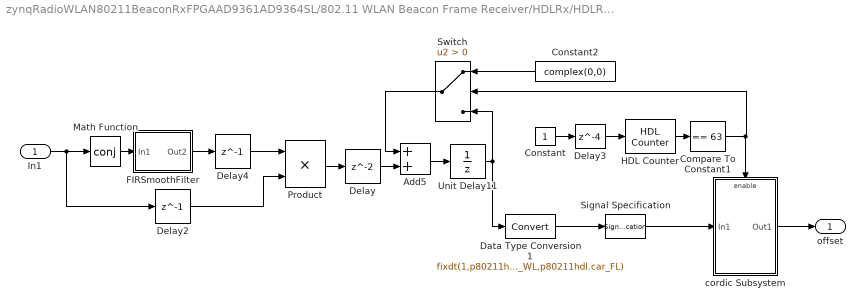
== system zynqRadioWLAN80211BeaconRxFPGAAD9361AD9364SL/802.11 WLAN Beacon Frame Receiver/HDLRx/HDLRx Front End/Coarse Frequency Compensation/luise_fixpt ==
  In1 : Inport
  Add5 : Sum  OutDataTypeStr=fixdt(1,p80211hdl.car_WL,p80211hdl.car_FL)  RndMeth=Nearest  SaturateOnIntegerOverflow=on
  Compare To Constant1 : simulink/Logic and Bit Operations/Compare To Constant  relop===  const=63  OutDataTypeStr=boolean
  Constant : Constant  OutDataTypeStr=boolean  SampleTime=-1
  Constant2 : Constant  Value=complex(0,0)  VectorParams1D=off  OutDataTypeStr=fixdt(1,p80211hdl.car_WL,p80211hdl.car_FL)  SampleTime=-1
  Data Type Conversion1 : DataTypeConversion  OutDataTypeStr=fixdt(1,p80211hdl.car_WL,p80211hdl.car_FL)  RndMeth=Nearest  SaturateOnIntegerOverflow=on
  Delay : Delay  InitialCondition=0
  Delay2 : Delay  DelayLength=1  InitialCondition=0
  Delay3 : Delay  DelayLength=4  InitialCondition=0
  Delay4 : Delay  DelayLength=1  InitialCondition=0
  FIRSmoothFilter : Subsystem
  HDL Counter : hdlsllib/HDL Operations/HDL Counter  CountType=Count limited  CountInit=0  CountStep=1  CountMax=63  CountFromType=Initial value  CountFrom=0  CountResetPort=off  CountLoadPort=off  CountEnbPort=on  CountDirPort=off  CountDataType=Unsigned  CountWordLen=6  CountFracLen=0  CountSampTime=-1
  Math Function : Math  Operator=conj  SaturateOnIntegerOverflow=on
  Product : Product  OutDataTypeStr=fixdt(1,p80211hdl.car_WL,p80211hdl.car_FL)  RndMeth=Nearest  SaturateOnIntegerOverflow=on
  Signal Specification : SignalSpecification  Dimensions=1
  Switch : Switch  Criteria=u2 > Threshold
  Unit Delay11 : UnitDelay  SampleTime=-1
  cordic Subsystem : Subsystem  TreatAsAtomicUnit=on
  offset : Outport  PortDimensions=1
  wires:
  cordic Subsystem/1(Out1) -> offset/1
  Data Type Conversion1/1 -> Signal Specification/1
  Compare To Constant1/1 -> Switch/2, cordic Subsystem/Enable
  HDL Counter/1 -> Compare To Constant1/1
  Add5/1 -> Unit Delay11/1
  Constant2/1 -> Switch/1
  Math Function/1 -> FIRSmoothFilter/1(In1)
  Unit Delay11/1 -> Data Type Conversion1/1, Switch/3
  FIRSmoothFilter/1(Out2) -> Delay4/1
  Product/1 -> Delay/1
  Delay/1 -> Add5/2
  Switch/1 -> Add5/1
  Delay4/1 -> Product/1
  Delay2/1 -> Product/2
  Constant/1 -> Delay3/1
  Delay3/1 -> HDL Counter/1
  In1/1 -> Math Function/1, Delay2/1
  Signal Specification/1 -> cordic Subsystem/1(In1)

== system zynqRadioWLAN80211BeaconRxFPGAAD9361AD9364SL/802.11 WLAN Beacon Frame Receiver/HDLRx/HDLRx Front End/Coarse Frequency Compensation/luise_fixpt/FIRSmoothFilter ==
  In1 : Inport
  Delay{,1..3} (4 alike) : Delay  DelayLength=1  InitialCondition=0
  ShiftArith : ArithShift  BitShiftNumber=6  BitShiftDirection=Right
  Sum : Sum  Inputs=|++  OutDataTypeStr=fixdt(1,16,5)  SaturateOnIntegerOverflow=on
  Sum1 : Sum  Inputs=|++  OutDataTypeStr=fixdt(1,16,5)  SaturateOnIntegerOverflow=on
  Sum2 : Sum  Inputs=|++  OutDataTypeStr=fixdt(1,16,4)  SaturateOnIntegerOverflow=on
  Out2 : Outport
  wires:
  In1/1 -> Delay/1
  Delay2/1 -> Sum1/1, Delay3/1
  Delay1/1 -> Sum/2, Delay2/1
  Delay/1 -> Sum/1, Delay1/1
  Sum/1 -> Sum2/1
  Sum1/1 -> Sum2/2
  Sum2/1 -> ShiftArith/1
  Delay3/1 -> Sum1/2
  ShiftArith/1 -> Out2/1

== system zynqRadioWLAN80211BeaconRxFPGAAD9361AD9364SL/802.11 WLAN Beacon Frame Receiver/HDLRx/HDLRx Front End/Coarse Frequency Compensation/luise_fixpt/cordic Subsystem ==
  In1 : Inport
  Enable : EnablePort
  Complex to Magnitude-Angle HDL Optimized : dspmathops/Complex to Magnitude-Angle HDL Optimized  NumIterationsSource=Property  NumIterations=5  OutputFormat=Angle  AngleFormat=Normalized  ScaleOutput=on  SimulateUsing=Code generation
  Constant : Constant  Value=p80211hdl.pInc_const  OutDataTypeStr=uint16  SampleTime=-1
  Constant1 : Constant  OutDataTypeStr=boolean  SampleTime=-1
  Product : Product  OutDataTypeStr=int16
  Terminator : Terminator
  Out1 : Outport  InitialOutput=0
  wires:
  Complex to Magnitude-Angle HDL Optimized/2 -> Terminator/1
  Constant1/1 -> Complex to Magnitude-Angle HDL Optimized/2
  In1/1 -> Complex to Magnitude-Angle HDL Optimized/1
  Complex to Magnitude-Angle HDL Optimized/1 -> Product/1
  Constant/1 -> Product/2
  Product/1 -> Out1/1

== matlab function zynqRadioWLAN80211BeaconRxFPGAAD9361AD9364SL/802.11 WLAN Beacon Frame Receiver/Detector/Packet Decoder/MPDU Decoder ==
  data: mpduCRC output; plcpCRC input boolean size=1; expLen input size=1; actLen input; payload input; mpdu output Bus: BeaconMPDUType size=[1 1]; detected output
function [mpduCRC, mpdu,detected] = mpduDec(plcpCRC, expLen, actLen, payload)
%#codegen

coder.extrinsic('warning')

persistent hCRC firstTime lastMPDU lastMpduCRC 

% Frame check sequence (FCS)
if isempty(hCRC)
  hCRC = comm.CRCDetector([32 26 23 22 16 12 11 10 8 7 5 4 2 1 0], ...
    'InitialConditions', 1, ...
    'DirectMethod',      true, ...
    'FinalXOR',          1);
  firstTime = true;
  lastMPDU.Header = parseMPDUHeader(zeros(64,1), 1);
  lastMPDU.FrameBody = unknownMPDU();
  lastMpduCRC = true;  % CRC is not zero
 
end

% If the CRC for the header decodes correctly (i.e. CRC flag is 0) and the
% received MPDU payload length is greater than or equal to the expected
% length, then turn on the MPDU decoder
detected = false;
if ~plcpCRC && (expLen > 0) && (actLen >= expLen) && (expLen >= 32) ...
    && firstTime
  % Compute CRC based on IEEE Std 802.11(TM)-2007 section 7.1.3.7.
  frameCRC = payload(1:expLen);
  [frame, mpduCRC] = step(hCRC, frameCRC);
  
  [mpdu.Header, mpduHeaderLen] = parseMPDUHeader(frame, mpduCRC);

  
  if (mpduCRC == 1) || ((mpdu.Header.FrameCtrl.Type ~= 0) ...
      || (mpdu.Header.FrameCtrl.Subtype ~= 8))
    mpdu.FrameBody = unknownMPDU();
   else
    mpdu.FrameBody = parseBeaconMPDU(frame(mpduHeaderLen+1:end, 1), mpduCRC);
    detected = true;
  end
  
  lastMPDU = mpdu;
  lastMpduCRC = mpduCRC;
  firstTime = false;
else
  mpdu = lastMPDU;
  mpduCRC = lastMpduCRC;
end

end

function [mpduHeader, len] = parseMPDUHeader(frame, mpduCRC)
% Based on IEEE Std 802.11-2007 chapter 7.

mpduHeader.FrameCtrl       = parseFrameControl(frame(1:16,1), mpduCRC);
mpduHeader.DurationID      = zeros(1,2,'uint8');
mpduHeader.Address1        = zeros(1,6,'uint8');
mpduHeader.Address2        = zeros(1,6,'uint8');
mpduHeader.Address3        = zeros(1,6,'uint8');
mpduHeader.SequenceControl = zeros(1,2,'uint8');
mpduHeader.Address4        = zeros(1,6,'uint8');
len = (2+6+6+6+2+6)*8 + 16;

if (mpduCRC == 0)
  p = 1;
  mpduHeader.FrameCtrl       = parseFrameControl(frame(p:p+15,1), mpduCRC);
  p = p+16;
  mpduHeader.DurationID      = bit2Octet(frame(p:p+15,1),2);
  p = p+16;
  mpduHeader.Address1        = bit2Octet(frame(p:p+47,1),6);
  p = p+48;
  
  isManagementFrame = (mpduHeader.FrameCtrl.Type == 0);
  isControlFrame = (mpduHeader.FrameCtrl.Type == 1);
  isDataFrame = (mpduHeader.FrameCtrl.Type == 2);
  isCTSFrame = isControlFrame && (mpduHeader.FrameCtrl.Subtype == 12);
  isACKFrame = isControlFrame && (mpduHeader.FrameCtrl.Subtype == 13);
  
  if ~(isCTSFrame || isACKFrame)
    mpduHeader.Address2        = bit2Octet(frame(p:p+47,1),6);
    p = p+48;
  end
  if isManagementFrame 
    mpduHeader.Address3        = bit2Octet(frame(p:p+47,1),6);
    p = p+48;
  end
  if ~isControlFrame
    mpduHeader.SequenceControl = bit2Octet(frame(p:p+15,1),2);
    p = p+16;
  end
  if isDataFrame
    mpduHeader.Address4        = bit2Octet(frame(p:p+47,1),6);
    p = p+48;
  end
  len = p-1;
end
end

function frameCtrl = parseFrameControl(fcBits, mpduCRC)
if (mpduCRC == 0)
  frameCtrl.ProtocolVersion = uint8(bi2de(fcBits(1:2,1)'));
  frameCtrl.Type            = uint8(bi2de(fcBits(3:4,1)'));
  frameCtrl.Subtype         = uint8(bi2de(fcBits(5:8,1)'));
  frameCtrl.ToDS            = uint8(bi2de(fcBits(9,1)'));
  frameCtrl.FromDS          = uint8(bi2de(fcBits(10,1)'));
  frameCtrl.MoreFragments   = uint8(bi2de(fcBits(11,1)'));
  frameCtrl.Retry           = uint8(bi2de(fcBits(12,1)'));
  frameCtrl.PowerManagement = uint8(bi2de(fcBits(13,1)'));
  frameCtrl.MoreData        = uint8(bi2de(fcBits(14,1)'));
  frameCtrl.ProtectedFrame  = uint8(bi2de(fcBits(15,1)'));
  frameCtrl.Order           = uint8(bi2de(fcBits(16,1)'));
else
  frameCtrl.ProtocolVersion = uint8(0);
  frameCtrl.Type            = uint8(0);
  frameCtrl.Subtype         = uint8(0);
  frameCtrl.ToDS            = uint8(0);
  frameCtrl.FromDS          = uint8(0);
  frameCtrl.MoreFragments   = uint8(0);
  frameCtrl.Retry           = uint8(0);
  frameCtrl.PowerManagement = uint8(0);
  frameCtrl.MoreData        = uint8(0);
  frameCtrl.ProtectedFrame  = uint8(0);
  frameCtrl.Order           = uint8(0);
end
end

function frameBody = parseBeaconMPDU(frame, mpduCRC)
if (mpduCRC == 0)
  bitCount = uint32(1);
  frameBody.TimeStamp      = bit2Octet(frame(bitCount:bitCount+63,1),8);
  bitCount = bitCount + 64;
  frameBody.BeaconInterval = bit2Octet(frame(bitCount:bitCount+15,1),2);
  bitCount = bitCount + 16;
  frameBody.Capability     = parseCapabilities(frame(81:96), mpduCRC);
  bitCount = bitCount + 16;
else
  frameBody.TimeStamp      = zeros(1,8,'uint8');
  frameBody.BeaconInterval = zeros(1,2,'uint8');
  frameBody.Capability     = parseCapabilities(frame(81:96), mpduCRC);
  bitCount = uint32(97);
end

frameLength = length(frame);

frameBody.NumInfoElements = uint8(0);
macElementStruct = struct('ID', uint8(255), ...
  'Length', uint8(0), ...
  'Value', zeros(1,257,'uint8'));
frameBody.InfoElements = repmat(macElementStruct, 1, 60);

if (mpduCRC == 0)
  while bitCount < frameLength
    frameBody.NumInfoElements = frameBody.NumInfoElements + 1;
    frameBody.InfoElements(frameBody.NumInfoElements).ID = ...
      bit2Octet(frame(bitCount:bitCount+7,1), 1);
    bitCount = bitCount + 8;
    elemLength = bit2Octet(frame(bitCount:bitCount+7,1), 1);
    frameBody.InfoElements(frameBody.NumInfoElements).Length = elemLength;
    bitCount = bitCount + 8;
    for p=1:elemLength
      frameBody.InfoElements(frameBody.NumInfoElements).Value(p) = ...
        bit2Octet(frame(bitCount:bitCount+7),1);
      bitCount = bitCount+8;
    end
  end
end
end

function capability = parseCapabilities(frame, mpduCRC)
if (mpduCRC == 0)
  capability.ESS                = frame(1,1);
  capability.IBSS               = frame(2,1);
  capability.CFPollable         = frame(3,1);
  capability.CFPollRequest      = frame(4,1);
  capability.Privacy            = frame(5,1);
  capability.ShortPreamble      = frame(6,1);
  capability.PBCC               = frame(7,1);
  capability.ChannelAgility     = frame(8,1);
  capability.SpectrumManagement = frame(9,1);
  capability.QoS                = frame(10,1);
  capability.ShortSlotTime      = frame(11,1);
  capability.APSD               = frame(12,1);
  capability.Reserved           = frame(13,1);
  capability.DSSOFDM            = frame(14,1);
  capability.DelayedBlockAck    = frame(15,1);
  capability.ImmediateBlockAck  = frame(16,1);
else
  capability.ESS                = false;
  capability.IBSS               = false;
  capability.CFPollable         = false;
  capability.CFPollRequest      = false;
  capability.Privacy            = false;
  capability.ShortPreamble      = false;
  capability.PBCC               = false;
  capability.ChannelAgility     = false;
  capability.SpectrumManagement = false;
  capability.QoS                = false;
  capability.ShortSlotTime      = false;
  capability.APSD               = false;
  capability.Reserved           = false;
  capability.DSSOFDM            = false;
  capability.DelayedBlockAck    = false;
  capability.ImmediateBlockAck  = false;
end
end

function frameBody = unknownMPDU()
frameBody.TimeStamp      = zeros(1,8,'uint8');
frameBody.BeaconInterval = zeros(1,2,'uint8');
frameBody.Capability     = parseCapabilities(zeros(16,1), 1);

frameBody.NumInfoElements = uint8(0);
macElementStruct = struct('ID', uint8(255), ...
  'Length', uint8(0), ...
  'Value', zeros(1,257,'uint8'));
frameBody.InfoElements = repmat(macElementStruct, 1, 60);
end

function octets = bit2Octet(bits,numOctets)
octets = zeros(1, numOctets, 'uint8');
for p=1:numOctets
  octets(1,p) = (bits((p-1)*8+1:p*8)')*2.^(0:7)';
end
end

== matlab function zynqRadioWLAN80211BeaconRxFPGAAD9361AD9364SL/802.11 WLAN Beacon Frame Receiver/Detector/Packet Decoder/Received MPDU/Received MPDU GUI ==
  data: plcpCRC input; mpduCRC input; mpdu input; OpenScopeAtSimStart parameter size=[1 1]; figPosition parameter
function mpduGUI(plcpCRC, mpduCRC, mpdu, OpenScopeAtSimStart, figPosition)
%#codegen

persistent resetGUI

if isempty(resetGUI)
  resetGUI = true;
end

coder.extrinsic('receivedFullMPDUGUI')

receivedFullMPDUGUI(mpdu.Header, mpdu.FrameBody, plcpCRC, mpduCRC, ...
  resetGUI, OpenScopeAtSimStart, figPosition);

resetGUI = false;

== matlab function zynqRadioWLAN80211BeaconRxFPGAAD9361AD9364SL/802.11 WLAN Beacon Frame Receiver/Beacon Counter/MATLAB Function ==
  data: numBeacon output; beaconflag input
function numBeacon   = fcn(beaconflag)


%#codegen


persistent   beaconcnt

if isempty (beaconcnt)
    beaconcnt = 0;
    
end

if beaconflag
    
    beaconcnt = beaconcnt+1;
    
end

numBeacon = beaconcnt;

== matlab function zynqRadioWLAN80211BeaconRxFPGAAD9361AD9364SL/802.11 WLAN Beacon Frame Receiver/HDLRx/HDLRx Controller/Rx Controller ==
  data: corrPeakVal input; corrPeakIdx input; startRx output; p80211 parameter; despreadSel output; p80211hdl parameter
function [startRx,despreadSel]  = rxCtrl(corrPeakVal, corrPeakIdx,p80211,p80211hdl)
%#codegen

persistent rxOn controllerState sampleCount lastSyncDelay

% State Enums
SearchPLCP = fi(0,0,1,0);
%WaitForSFD = 1;
GetSamples = fi(1,0,1,0);

if isempty(rxOn)
  % Initialize receiver controller
  rxOn = false;
  controllerState = SearchPLCP;
  sampleCount   = fi(0,0,17,0);
  lastSyncDelay = uint8(1);
end

switch controllerState
  case SearchPLCP,
    if corrPeakVal > p80211.CorrelationThreshold % 1500
      % Synchronize to the end of the SYNC. Get 8 (scrambler length) extra
      % bits to initialize DPSK demodulator and scrambler
      scramblerLen = length(p80211.ScramblerPolynomial);
%       lastSyncDelay = p80211.SamplesPerChannelFrame - (corrPeakIdx);% ...
%         - scramblerLen*p80211.SpreadingRate*p80211.SamplesPerChip); 
       lastSyncDelay = corrPeakIdx;
      %sampleCount(1) = p80211.NumSYNCSamples ...
       % - scramblerLen*p80211.SpreadingRate*p80211.SamplesPerChip;
       sampleCount(1) = p80211.SymbolsPerChannelFrame - scramblerLen;
       %sampleCount.data = (countval, 0, 17,0);
      rxOn = true;
      
      controllerState = GetSamples;
    end
%   case WaitForSFD
%       rxOn = true;
%       controllerState = GetSamples;
  case GetSamples
    % In this state we recevie both SFD, which is part of PLCP preamble,
    % the PLCP header, and MPDU.
    
    sampleCount(1) = sampleCount + fi(1,0,17,0);
    
    if  (sampleCount(1) >= p80211hdl.dataCount)
        %(sampleCount >= (p80211.NumPLCPSamples+...
        %p80211.ScramblerAmbiguitySamples+p80211.MaximumPayloadSamples))/22;
        
      rxOn = false;
      lastSyncDelay = uint8(1);
    %despreadSel = 1;
      controllerState = SearchPLCP;
    end
end

startRx = rxOn;
despreadSel =  lastSyncDelay;
% syncDelay = lastSyncDelay;
